simulink library "SkywardBLIMP"  (R2015a)
settings: Solver=ode45  StartTime=0.0  StopTime=10.0  RelTol=1e-3
settings Model: Creator=Francescodario  LastModifiedBy=franc

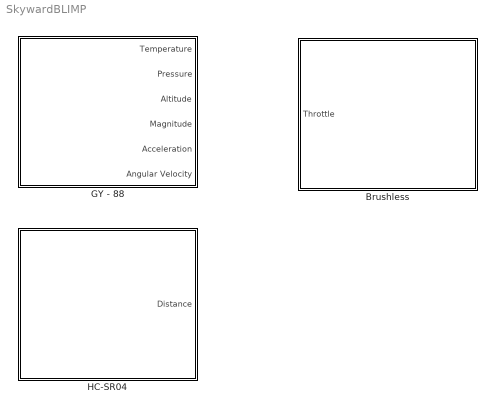
== system SkywardBLIMP ==
  Brushless : Subsystem  mask{PIN=9, S_T=0.01}
      mask prompts: S_T "Sample Time"
      mask help:
      | This block drive the Brushless motors of the BLIMP. Please do not modify the internal subsystem
      | parameters.
      mask Display:
      | %Load the image
      | rgb = imread('blocks\ESC\ESC.jpg');
      | % Display the image
      | image(rgb);
      | port_label('input',1,'Throttle')
  "GY - 88 " : Subsystem  mask(GY-88){S_T=0.02}
      mask prompts: S_T "Sample Time"
      mask help:
      | This block will output data from GY-88 IMU. Magnitude, Acceleration and Angular Velocity are
      | given as 3 components vectors.
      mask Display:
      | %Load the image
      | rgb = imread('blocks\GY-88\GY-88.jpg');
      | % Display the image
      | image(rgb);
      | %Port labels
      | port_label('output',1,'Temperature')
      | port_label('output',2,'Pressure')
      | port_label('output',3,'Altitude')
      | port_label('output',4,'Magnitude')
      | port_label('output',5,'Acceleration')
      | port_label('output',6,'Angular Velocity')
  HC-SR04 : Subsystem  mask{S_T=0.02}
      mask prompts: S_T "Sample Time"
      mask help:
      | This block drive the HC-SR04 ultrasonic sensor.
      | The Trig PIN should be connected to Arduino PIN 3, the Echo PIN should be
      | connected to Arduino PIN 2.
      mask Display:
      | %Load the image
      | rgb = imread('blocks\HC-SR04\HC-SR04.jpg');
      | % Display the image
      | image(rgb);
      | port_label('output',1,'Distance')

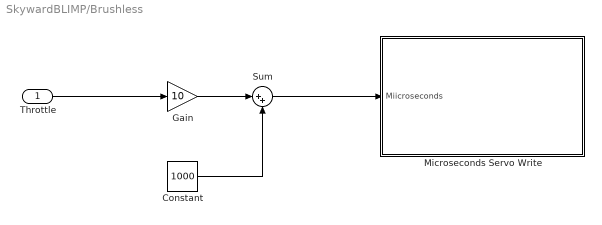
== system SkywardBLIMP/Brushless ==
  Throttle : Inport
  Constant : Constant  Value=1000
  Gain : Gain  Gain=10
  Microseconds Servo Write : Subsystem  mask{S_T=S_T, PIN=PIN}
      mask prompts: S_T "Sample Time"
  Sum : Sum  Inputs=|++
  wires:
  Constant/1 -> Sum/2
  Sum/1 -> Microseconds Servo Write/1("Miicroseconds ")
  Throttle/1 -> Gain/1
  Gain/1 -> Sum/1

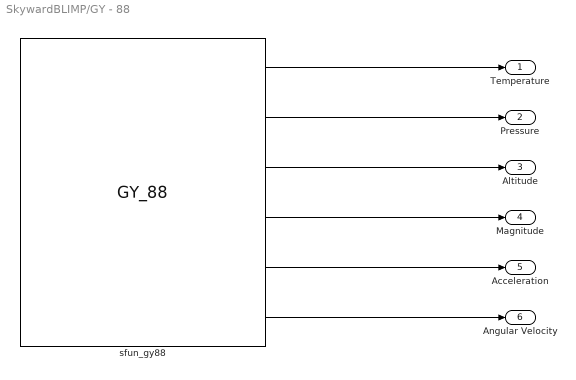
== system SkywardBLIMP/GY - 88  ==
  sfun_gy88 : S-Function  FunctionName=GY_88  Parameters=1  SFunctionModules='GY_88 GY_88_wrapper'
  Temperature : Outport
  Pressure : Outport  Port=2
  Altitude : Outport  Port=3
  Magnitude : Outport  Port=4
  Acceleration : Outport  Port=5
  Angular Velocity : Outport  Port=6
  wires:
  sfun_gy88/5 -> Acceleration/1
  sfun_gy88/3 -> Altitude/1
  sfun_gy88/6 -> Angular Velocity/1
  sfun_gy88/2 -> Pressure/1
  sfun_gy88/4 -> Magnitude/1
  sfun_gy88/1 -> Temperature/1

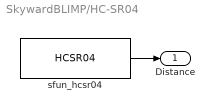
== system SkywardBLIMP/HC-SR04 ==
  sfun_hcsr04 : S-Function  FunctionName=HCSR04  Parameters=1  SFunctionModules='HCSR04 HCSR04_wrapper'
  "Distance " : Outport
  wires:
  sfun_hcsr04/1 -> "Distance "/1

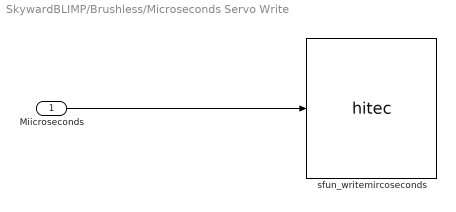
== system SkywardBLIMP/Brushless/Microseconds Servo Write ==
  "Miicroseconds " : Inport
  sfun_writemircoseconds : S-Function  FunctionName=hitec  Parameters=2,2  SFunctionModules='hitec hitec_wrapper'
  wires:
  "Miicroseconds "/1 -> sfun_writemircoseconds/1
